simulink model "Excavator_Complete"  (R2026a)
settings: Solver=ode23t  StopTime=stopTime  MaxStep=Ts  AbsTol=1e-3
PostLoadFcn:
  | set_param(bdroot,'IgnoredZcDiagnostic','none');
  | Excavator_Test_Scenario_Select('loadedBucketDigCycle');
model workspace: external: MAT-File ExcavatorAssemblyDataStruct.mat (data not in the file)
undefined symbols (not defined in the file or in its folder): AToBRegOrificeVector, AToTOrificeVector, BiPOrificeVector, BoomC, boomHEArea, boomREArea, boomUpMaxQ, boomValve, BToTOrificeVector, BucketC, bucketCloseMaxQ, bucketOpenMaxQ, BucketR, bucketValve, fluids, gravity, LeftBoomR, materialWeight, maxPumpDisp, minPumpDisp, nominalEngineSpeed, P28Assembly, PToAOrificeVector, PToBOrificeVector, pumpCmdNegRateLimit, pumpCmdPosRateLimit, RightBoomR, startDiggingZPos, StickC, stickInMaxQ, stickOutMaxQ, StickR, stickValve, SwingC, swingDisplacement, swingHighSpeedThreshold, swingMaxQ, SwingR, swingSpeedQGain, swingValve, valveCmdNegRateLimit, valveCmdPosRateLimit, velocityToYForceGain, X, Y, yForceMax, yForceToZForceGain, Z, zForceMax
libraries: fl_lib x89, sm_lib x80, SimscapeFluids_lib x78, nesl_utility x50, simulink_extras x11, Excavator_Parts_Lib x6, simulink x2, SignalEditorBlockLib x1
(part 7 of 7)

== system Excavator_Complete/Excavator/Hydraulics/ValveBlocks/RightValveBlock/Bucket Valve ==
  AtoT : SimscapeFluids_lib/Isothermal Liquid/Valves & Orifices/Orifices/Orifice (IL)  orifice_type=foundation.enum.constant_variable.variable  constant_orifice_spec=fluids.isothermal_liquid.valves_orifices.orifices.enum.constant_orifice_spec.area  variable_orifice_spec=fluids.isothermal_liquid.valves_orifices.orifices.enum.orifice_spec.table1D_area_opening  orifice_area_constant=1e-3 m^2  p_diff_TLU_constant=[-4, -3, -2, -1, -.5, 0, .5, 1, 2, 3, 4] MPa  vol_flow_TLU_constant=[-2.44, -2.12, -1.68, -1.22, -.84, 0, .85, 1.21, 1.7, 2.09, 2.41] .* 1e-3 m^3/s  S_min=1e-10 m  del_S=0.005 m  open_orientation=fluids.isothermal_liquid.valves_orifices.orifices.enum.orifice_orientation.positive  area_max=0.5e-4 m^2  area_leak=1e-12 m^2  S_TLU=valveData.spoolPosVector mm  orifice_area_TLU=valveData.AtoTOrificeAreaVector mm^2  area=inf m^2  Cd=0.7  Re_c=150  smoothing_factor=0  pressure_recovery=simscape.enum.onoff.off  S_vol_flow_TLU=AToTOrificeVector - 1000*(0) mm  p_diff_TLU=[-10000000, -5000000, -2000000, 2000000, 5000000, 10000000] Pa  vol_flow_TLU=[-1e-07, -7.0711e-08, -4.4721e-08, 4.4721e-08, 7.0711e-08, 1e-07; -2.0352e-05, -1.4391e-05, -9.1017e-06, 9.1017e-06, 1.4391e-05, 2.0352e-05; -.0040736, -.0028805, -.0018218, .0018218, .0028805, .0040736; -.011438, -.0080879, -.0051152, .0051152, .0080879, .011438; -.034356, -.024293, -.015364, .015364, .024293, .034356] m^3/s
  BiPOrifice : SimscapeFluids_lib/Isothermal Liquid/Valves & Orifices/Orifices/Orifice (IL)  orifice_type=foundation.enum.constant_variable.variable  constant_orifice_spec=fluids.isothermal_liquid.valves_orifices.orifices.enum.constant_orifice_spec.area  variable_orifice_spec=fluids.isothermal_liquid.valves_orifices.orifices.enum.orifice_spec.table1D_area_opening  orifice_area_constant=1e-3 m^2  p_diff_TLU_constant=[-4, -3, -2, -1, -.5, 0, .5, 1, 2, 3, 4] MPa  vol_flow_TLU_constant=[-2.44, -2.12, -1.68, -1.22, -.84, 0, .85, 1.21, 1.7, 2.09, 2.41] .* 1e-3 m^3/s  S_min=1e-10 m  del_S=0.005 m  open_orientation=fluids.isothermal_liquid.valves_orifices.orifices.enum.orifice_orientation.positive  area_max=0.5e-4 m^2  area_leak=1e-12 m^2  S_TLU=valveData.spoolPosVector mm  orifice_area_TLU=valveData.BiPOrificeAreaVector mm^2  area=inf m^2  Cd=0.7  Re_c=150  smoothing_factor=0  pressure_recovery=simscape.enum.onoff.off  S_vol_flow_TLU=BiPOrificeVector - 1000*(0) mm  p_diff_TLU=[-10000000, -5000000, -2000000, 2000000, 5000000, 10000000] Pa  vol_flow_TLU=[-1e-07, -7.0711e-08, -4.4721e-08, 4.4721e-08, 7.0711e-08, 1e-07; -2.0352e-05, -1.4391e-05, -9.1017e-06, 9.1017e-06, 1.4391e-05, 2.0352e-05; -.0040736, -.0028805, -.0018218, .0018218, .0028805, .0040736; -.011438, -.0080879, -.0051152, .0051152, .0080879, .011438; -.034356, -.024293, -.015364, .015364, .024293, .034356] m^3/s
  BtoT : SimscapeFluids_lib/Isothermal Liquid/Valves & Orifices/Orifices/Orifice (IL)  orifice_type=foundation.enum.constant_variable.variable  constant_orifice_spec=fluids.isothermal_liquid.valves_orifices.orifices.enum.constant_orifice_spec.area  variable_orifice_spec=fluids.isothermal_liquid.valves_orifices.orifices.enum.orifice_spec.table1D_area_opening  orifice_area_constant=1e-3 m^2  p_diff_TLU_constant=[-4, -3, -2, -1, -.5, 0, .5, 1, 2, 3, 4] MPa  vol_flow_TLU_constant=[-2.44, -2.12, -1.68, -1.22, -.84, 0, .85, 1.21, 1.7, 2.09, 2.41] .* 1e-3 m^3/s  S_min=1e-10 m  del_S=0.005 m  open_orientation=fluids.isothermal_liquid.valves_orifices.orifices.enum.orifice_orientation.positive  area_max=0.5e-4 m^2  area_leak=1e-12 m^2  S_TLU=valveData.spoolPosVector mm  orifice_area_TLU=valveData.BtoTOrificeAreaVector mm^2  area=inf m^2  Cd=0.7  Re_c=150  smoothing_factor=0  pressure_recovery=simscape.enum.onoff.off  S_vol_flow_TLU=BToTOrificeVector - 1000*(0) mm  p_diff_TLU=[-10000000, -5000000, -2000000, 2000000, 5000000, 10000000] Pa  vol_flow_TLU=[-1e-07, -7.0711e-08, -4.4721e-08, 4.4721e-08, 7.0711e-08, 1e-07; -2.0352e-05, -1.4391e-05, -9.1017e-06, 9.1017e-06, 1.4391e-05, 2.0352e-05; -.0040736, -.0028805, -.0018218, .0018218, .0028805, .0040736; -.011438, -.0080879, -.0051152, .0051152, .0080879, .011438; -.034356, -.024293, -.015364, .015364, .024293, .034356] m^3/s
  PS Abs : fl_lib/Physical Signals/Nonlinear Operators/PS Abs  ZeroCross=true
  PS Gain1 : fl_lib/Physical Signals/Functions/PS Gain  gain=-1
  PtoA : SimscapeFluids_lib/Isothermal Liquid/Valves & Orifices/Orifices/Orifice (IL)  orifice_type=foundation.enum.constant_variable.variable  constant_orifice_spec=fluids.isothermal_liquid.valves_orifices.orifices.enum.constant_orifice_spec.area  variable_orifice_spec=fluids.isothermal_liquid.valves_orifices.orifices.enum.orifice_spec.table1D_area_opening  orifice_area_constant=1e-3 m^2  p_diff_TLU_constant=[-4, -3, -2, -1, -.5, 0, .5, 1, 2, 3, 4] MPa  vol_flow_TLU_constant=[-2.44, -2.12, -1.68, -1.22, -.84, 0, .85, 1.21, 1.7, 2.09, 2.41] .* 1e-3 m^3/s  S_min=1e-10 m  del_S=0.005 m  open_orientation=fluids.isothermal_liquid.valves_orifices.orifices.enum.orifice_orientation.positive  area_max=0.5e-4 m^2  area_leak=1e-12 m^2  S_TLU=valveData.spoolPosVector mm  orifice_area_TLU=valveData.PtoAOrificeAreaVector mm^2  area=inf m^2  Cd=0.7  Re_c=150  smoothing_factor=0  pressure_recovery=simscape.enum.onoff.off  S_vol_flow_TLU=PToAOrificeVector - 1000*(0) mm  p_diff_TLU=[-10000000, -5000000, -2000000, 2000000, 5000000, 10000000] Pa  vol_flow_TLU=[-1e-07, -7.0711e-08, -4.4721e-08, 4.4721e-08, 7.0711e-08, 1e-07; -2.0352e-05, -1.4391e-05, -9.1017e-06, 9.1017e-06, 1.4391e-05, 2.0352e-05; -.0040736, -.0028805, -.0018218, .0018218, .0028805, .0040736; -.011438, -.0080879, -.0051152, .0051152, .0080879, .011438; -.034356, -.024293, -.015364, .015364, .024293, .034356] m^3/s
  PtoB : SimscapeFluids_lib/Isothermal Liquid/Valves & Orifices/Orifices/Orifice (IL)  orifice_type=foundation.enum.constant_variable.variable  constant_orifice_spec=fluids.isothermal_liquid.valves_orifices.orifices.enum.constant_orifice_spec.area  variable_orifice_spec=fluids.isothermal_liquid.valves_orifices.orifices.enum.orifice_spec.table1D_area_opening  orifice_area_constant=1e-3 m^2  p_diff_TLU_constant=[-4, -3, -2, -1, -.5, 0, .5, 1, 2, 3, 4] MPa  vol_flow_TLU_constant=[-2.44, -2.12, -1.68, -1.22, -.84, 0, .85, 1.21, 1.7, 2.09, 2.41] .* 1e-3 m^3/s  S_min=1e-10 m  del_S=0.005 m  open_orientation=fluids.isothermal_liquid.valves_orifices.orifices.enum.orifice_orientation.positive  area_max=0.5e-4 m^2  area_leak=1e-12 m^2  S_TLU=valveData.spoolPosVector mm  orifice_area_TLU=valveData.PtoBOrificeAreaVector mm^2  area=inf m^2  Cd=0.7  Re_c=150  smoothing_factor=0  pressure_recovery=simscape.enum.onoff.off  S_vol_flow_TLU=PToBOrificeVector - 1000*(0) mm  p_diff_TLU=[-10000000, -5000000, -2000000, 2000000, 5000000, 10000000] Pa  vol_flow_TLU=[-1e-07, -7.0711e-08, -4.4721e-08, 4.4721e-08, 7.0711e-08, 1e-07; -2.0352e-05, -1.4391e-05, -9.1017e-06, 9.1017e-06, 1.4391e-05, 2.0352e-05; -.0040736, -.0028805, -.0018218, .0018218, .0028805, .0040736; -.011438, -.0080879, -.0051152, .0051152, .0080879, .011438; -.034356, -.024293, -.015364, .015364, .024293, .034356] m^3/s
  S : PMIOPort  Side=Left
  P : PMIOPort  Port=2  Side=Left
  T : PMIOPort  Port=3  Side=Left
  BiPIn : PMIOPort  Port=4  Side=Left
  A : PMIOPort  Port=5  Side=Right
  B : PMIOPort  Port=6  Side=Right
  BiPOut : PMIOPort  Port=7  Side=Right
  connections:
  BtoT/LConn2 -- PtoA/LConn2 -- PS Gain1/RConn1
  BiPOrifice/LConn2 -- PS Abs/RConn1
  S/RConn1 -- PtoB/LConn2 -- AtoT/LConn2 -- PS Gain1/LConn1 -- PS Abs/LConn1
  T/RConn1 -- BtoT/RConn1 -- AtoT/RConn1
  BiPOrifice/RConn1 -- BiPOut/RConn1
  BiPOrifice/LConn1 -- BiPIn/RConn1
  PtoA/RConn1 -- A/RConn1 -- AtoT/LConn1
  PtoB/LConn1 -- P/RConn1 -- PtoA/LConn1
  PtoB/RConn1 -- BtoT/LConn1 -- B/RConn1

== system Excavator_Complete/Excavator/Hydraulics/ValveBlocks/RightValveBlock/Cmd to Spool Pos ==
  Cmds : Inport
  Bus Selector : BusSelector  OutputSignals=BMSpoolPos,SKSpoolPos,BTSpoolPos
  Simulink-PS Converter : nesl_utility/Simulink-PS Converter  PhysicalDomain=network_engine_domain  SubClassName=ps_input  LeftPortType=input  RightPortType=output  PseudoPeriodic=off  Frequencies=[]  NoiseDistribution=none  NoiseParameters=[]  Unit=mm  AffineConversion=off  FilteringAndDerivatives=provide  SimscapeFilterOrder=1  InputFilterTimeConstant=0.001  UdotUserProvided=0
  Simulink-PS Converter1 : nesl_utility/Simulink-PS Converter  PhysicalDomain=network_engine_domain  SubClassName=ps_input  LeftPortType=input  RightPortType=output  PseudoPeriodic=off  Frequencies=[]  NoiseDistribution=none  NoiseParameters=[]  Unit=mm  AffineConversion=off  FilteringAndDerivatives=provide  SimscapeFilterOrder=1  InputFilterTimeConstant=0.001  UdotUserProvided=0
  Simulink-PS Converter2 : nesl_utility/Simulink-PS Converter  PhysicalDomain=network_engine_domain  SubClassName=ps_input  LeftPortType=input  RightPortType=output  PseudoPeriodic=off  Frequencies=[]  NoiseDistribution=none  NoiseParameters=[]  Unit=mm  AffineConversion=off  FilteringAndDerivatives=provide  SimscapeFilterOrder=1  InputFilterTimeConstant=0.001  UdotUserProvided=0
  BMPos : PMIOPort  Side=Right
  SKPos : PMIOPort  Port=2  Side=Right
  BTPos : PMIOPort  Port=3  Side=Right
  wires:
  Bus Selector/1 -> Simulink-PS Converter/1  "<BMSpoolPos>"
  Bus Selector/3 -> Simulink-PS Converter2/1  "<BTSpoolPos>"
  Bus Selector/2 -> Simulink-PS Converter1/1  "<SKSpoolPos>"
  Cmds/1 -> Bus Selector/1
  connections:
  Simulink-PS Converter/RConn1 -- BMPos/RConn1
  Simulink-PS Converter1/RConn1 -- SKPos/RConn1
  Simulink-PS Converter2/RConn1 -- BTPos/RConn1

== system Excavator_Complete/Excavator/Hydraulics/ValveBlocks/RightValveBlock/Stick Valve ==
  AtoT : SimscapeFluids_lib/Isothermal Liquid/Valves & Orifices/Orifices/Orifice (IL)  orifice_type=foundation.enum.constant_variable.variable  constant_orifice_spec=fluids.isothermal_liquid.valves_orifices.orifices.enum.constant_orifice_spec.area  variable_orifice_spec=fluids.isothermal_liquid.valves_orifices.orifices.enum.orifice_spec.table1D_area_opening  orifice_area_constant=1e-3 m^2  p_diff_TLU_constant=[-4, -3, -2, -1, -.5, 0, .5, 1, 2, 3, 4] MPa  vol_flow_TLU_constant=[-2.44, -2.12, -1.68, -1.22, -.84, 0, .85, 1.21, 1.7, 2.09, 2.41] .* 1e-3 m^3/s  S_min=1e-10 m  del_S=0.005 m  open_orientation=fluids.isothermal_liquid.valves_orifices.orifices.enum.orifice_orientation.positive  area_max=0.5e-4 m^2  area_leak=1e-12 m^2  S_TLU=valveData.spoolPosVector mm  orifice_area_TLU=valveData.AtoTOrificeAreaVector mm^2  area=inf m^2  Cd=0.7  Re_c=150  smoothing_factor=0  pressure_recovery=simscape.enum.onoff.off  S_vol_flow_TLU=AToTOrificeVector - 1000*(0) mm  p_diff_TLU=[-10000000, -5000000, -2000000, 2000000, 5000000, 10000000] Pa  vol_flow_TLU=[-1e-07, -7.0711e-08, -4.4721e-08, 4.4721e-08, 7.0711e-08, 1e-07; -2.0352e-05, -1.4391e-05, -9.1017e-06, 9.1017e-06, 1.4391e-05, 2.0352e-05; -.0040736, -.0028805, -.0018218, .0018218, .0028805, .0040736; -.011438, -.0080879, -.0051152, .0051152, .0080879, .011438; -.034356, -.024293, -.015364, .015364, .024293, .034356] m^3/s
  BiPOrifice : SimscapeFluids_lib/Isothermal Liquid/Valves & Orifices/Orifices/Orifice (IL)  orifice_type=foundation.enum.constant_variable.variable  constant_orifice_spec=fluids.isothermal_liquid.valves_orifices.orifices.enum.constant_orifice_spec.area  variable_orifice_spec=fluids.isothermal_liquid.valves_orifices.orifices.enum.orifice_spec.table1D_area_opening  orifice_area_constant=1e-3 m^2  p_diff_TLU_constant=[-4, -3, -2, -1, -.5, 0, .5, 1, 2, 3, 4] MPa  vol_flow_TLU_constant=[-2.44, -2.12, -1.68, -1.22, -.84, 0, .85, 1.21, 1.7, 2.09, 2.41] .* 1e-3 m^3/s  S_min=1e-10 m  del_S=0.005 m  open_orientation=fluids.isothermal_liquid.valves_orifices.orifices.enum.orifice_orientation.positive  area_max=0.5e-4 m^2  area_leak=1e-12 m^2  S_TLU=valveData.spoolPosVector mm  orifice_area_TLU=valveData.BiPOrificeAreaVector mm^2  area=inf m^2  Cd=0.7  Re_c=150  smoothing_factor=0  pressure_recovery=simscape.enum.onoff.off  S_vol_flow_TLU=BiPOrificeVector - 1000*(0) mm  p_diff_TLU=[-10000000, -5000000, -2000000, 2000000, 5000000, 10000000] Pa  vol_flow_TLU=[-1e-07, -7.0711e-08, -4.4721e-08, 4.4721e-08, 7.0711e-08, 1e-07; -2.0352e-05, -1.4391e-05, -9.1017e-06, 9.1017e-06, 1.4391e-05, 2.0352e-05; -.0040736, -.0028805, -.0018218, .0018218, .0028805, .0040736; -.011438, -.0080879, -.0051152, .0051152, .0080879, .011438; -.034356, -.024293, -.015364, .015364, .024293, .034356] m^3/s
  BtoARegen : SimscapeFluids_lib/Isothermal Liquid/Valves & Orifices/Orifices/Orifice (IL)  orifice_type=foundation.enum.constant_variable.variable  constant_orifice_spec=fluids.isothermal_liquid.valves_orifices.orifices.enum.constant_orifice_spec.area  variable_orifice_spec=fluids.isothermal_liquid.valves_orifices.orifices.enum.orifice_spec.table1D_area_opening  orifice_area_constant=1e-3 m^2  p_diff_TLU_constant=[-4, -3, -2, -1, -.5, 0, .5, 1, 2, 3, 4] MPa  vol_flow_TLU_constant=[-2.44, -2.12, -1.68, -1.22, -.84, 0, .85, 1.21, 1.7, 2.09, 2.41] .* 1e-3 m^3/s  S_min=1e-10 m  del_S=0.005 m  open_orientation=fluids.isothermal_liquid.valves_orifices.orifices.enum.orifice_orientation.positive  area_max=0.5e-4 m^2  area_leak=1e-12 m^2  S_TLU=valveData.spoolPosVector mm  orifice_area_TLU=valveData.BtoARegOrificeAreaVector mm^2  area=inf m^2  Cd=0.7  Re_c=150  smoothing_factor=0  pressure_recovery=simscape.enum.onoff.off  S_vol_flow_TLU=AToBRegOrificeVector - 1000*(0) mm  p_diff_TLU=[-10000000, -5000000, -2000000, 2000000, 5000000, 10000000] Pa  vol_flow_TLU=[-1e-07, -7.0711e-08, -4.4721e-08, 4.4721e-08, 7.0711e-08, 1e-07; -2.0352e-05, -1.4391e-05, -9.1017e-06, 9.1017e-06, 1.4391e-05, 2.0352e-05; -.0040736, -.0028805, -.0018218, .0018218, .0028805, .0040736; -.011438, -.0080879, -.0051152, .0051152, .0080879, .011438; -.034356, -.024293, -.015364, .015364, .024293, .034356] m^3/s
  BtoT : SimscapeFluids_lib/Isothermal Liquid/Valves & Orifices/Orifices/Orifice (IL)  orifice_type=foundation.enum.constant_variable.variable  constant_orifice_spec=fluids.isothermal_liquid.valves_orifices.orifices.enum.constant_orifice_spec.area  variable_orifice_spec=fluids.isothermal_liquid.valves_orifices.orifices.enum.orifice_spec.table1D_area_opening  orifice_area_constant=1e-3 m^2  p_diff_TLU_constant=[-4, -3, -2, -1, -.5, 0, .5, 1, 2, 3, 4] MPa  vol_flow_TLU_constant=[-2.44, -2.12, -1.68, -1.22, -.84, 0, .85, 1.21, 1.7, 2.09, 2.41] .* 1e-3 m^3/s  S_min=1e-10 m  del_S=0.005 m  open_orientation=fluids.isothermal_liquid.valves_orifices.orifices.enum.orifice_orientation.positive  area_max=0.5e-4 m^2  area_leak=1e-12 m^2  S_TLU=valveData.spoolPosVector mm  orifice_area_TLU=valveData.BtoTOrificeAreaVector mm^2  area=inf m^2  Cd=0.7  Re_c=150  smoothing_factor=0  pressure_recovery=simscape.enum.onoff.off  S_vol_flow_TLU=BToTOrificeVector - 1000*(0) mm  p_diff_TLU=[-10000000, -5000000, -2000000, 2000000, 5000000, 10000000] Pa  vol_flow_TLU=[-1e-07, -7.0711e-08, -4.4721e-08, 4.4721e-08, 7.0711e-08, 1e-07; -2.0352e-05, -1.4391e-05, -9.1017e-06, 9.1017e-06, 1.4391e-05, 2.0352e-05; -.0040736, -.0028805, -.0018218, .0018218, .0028805, .0040736; -.011438, -.0080879, -.0051152, .0051152, .0080879, .011438; -.034356, -.024293, -.015364, .015364, .024293, .034356] m^3/s
  PS Abs : fl_lib/Physical Signals/Nonlinear Operators/PS Abs  ZeroCross=true
  PS Gain1 : fl_lib/Physical Signals/Functions/PS Gain  gain=-1
  PtoA : SimscapeFluids_lib/Isothermal Liquid/Valves & Orifices/Orifices/Orifice (IL)  orifice_type=foundation.enum.constant_variable.variable  constant_orifice_spec=fluids.isothermal_liquid.valves_orifices.orifices.enum.constant_orifice_spec.area  variable_orifice_spec=fluids.isothermal_liquid.valves_orifices.orifices.enum.orifice_spec.table1D_area_opening  orifice_area_constant=1e-3 m^2  p_diff_TLU_constant=[-4, -3, -2, -1, -.5, 0, .5, 1, 2, 3, 4] MPa  vol_flow_TLU_constant=[-2.44, -2.12, -1.68, -1.22, -.84, 0, .85, 1.21, 1.7, 2.09, 2.41] .* 1e-3 m^3/s  S_min=1e-10 m  del_S=0.005 m  open_orientation=fluids.isothermal_liquid.valves_orifices.orifices.enum.orifice_orientation.positive  area_max=0.5e-4 m^2  area_leak=1e-12 m^2  S_TLU=valveData.spoolPosVector mm  orifice_area_TLU=valveData.PtoAOrificeAreaVector mm^2  area=inf m^2  Cd=0.7  Re_c=150  smoothing_factor=0  pressure_recovery=simscape.enum.onoff.off  S_vol_flow_TLU=PToAOrificeVector - 1000*(0) mm  p_diff_TLU=[-10000000, -5000000, -2000000, 2000000, 5000000, 10000000] Pa  vol_flow_TLU=[-1e-07, -7.0711e-08, -4.4721e-08, 4.4721e-08, 7.0711e-08, 1e-07; -2.0352e-05, -1.4391e-05, -9.1017e-06, 9.1017e-06, 1.4391e-05, 2.0352e-05; -.0040736, -.0028805, -.0018218, .0018218, .0028805, .0040736; -.011438, -.0080879, -.0051152, .0051152, .0080879, .011438; -.034356, -.024293, -.015364, .015364, .024293, .034356] m^3/s
  PtoB : SimscapeFluids_lib/Isothermal Liquid/Valves & Orifices/Orifices/Orifice (IL)  orifice_type=foundation.enum.constant_variable.variable  constant_orifice_spec=fluids.isothermal_liquid.valves_orifices.orifices.enum.constant_orifice_spec.area  variable_orifice_spec=fluids.isothermal_liquid.valves_orifices.orifices.enum.orifice_spec.table1D_area_opening  orifice_area_constant=1e-3 m^2  p_diff_TLU_constant=[-4, -3, -2, -1, -.5, 0, .5, 1, 2, 3, 4] MPa  vol_flow_TLU_constant=[-2.44, -2.12, -1.68, -1.22, -.84, 0, .85, 1.21, 1.7, 2.09, 2.41] .* 1e-3 m^3/s  S_min=1e-10 m  del_S=0.005 m  open_orientation=fluids.isothermal_liquid.valves_orifices.orifices.enum.orifice_orientation.positive  area_max=0.5e-4 m^2  area_leak=1e-12 m^2  S_TLU=valveData.spoolPosVector mm  orifice_area_TLU=valveData.PtoBOrificeAreaVector mm^2  area=inf m^2  Cd=0.7  Re_c=150  smoothing_factor=0  pressure_recovery=simscape.enum.onoff.off  S_vol_flow_TLU=PToBOrificeVector - 1000*(0) mm  p_diff_TLU=[-10000000, -5000000, -2000000, 2000000, 5000000, 10000000] Pa  vol_flow_TLU=[-1e-07, -7.0711e-08, -4.4721e-08, 4.4721e-08, 7.0711e-08, 1e-07; -2.0352e-05, -1.4391e-05, -9.1017e-06, 9.1017e-06, 1.4391e-05, 2.0352e-05; -.0040736, -.0028805, -.0018218, .0018218, .0028805, .0040736; -.011438, -.0080879, -.0051152, .0051152, .0080879, .011438; -.034356, -.024293, -.015364, .015364, .024293, .034356] m^3/s
  StickRegenCV : SimscapeFluids_lib/Isothermal Liquid/Valves & Orifices/Directional Control Valves/Check Valve (IL)  opening_spec=2*(fluids.isothermal_liquid.valves_orifices.enum.opening_spec.linear)-1  pressure_control_spec=fluids.isothermal_liquid.valves_orifices.enum.pressure_control_spec.dp  p_crack_differential=valveData.checkValveCrackingPrDiff bar  p_crack_gauge=0.1 MPa  press_max_differential=valveData.checkValveMaxOpeningPrDiff bar  press_max_gauge=0.2 MPa  area_max=valveData.checkValveMaxOpeningArea mm^2  area_leak=valveData.checkValveLeakageArea mm^2  p_diff_TLU=[0.01 : 0.01 : 0.1] MPa  valve_area_TLU=[1e-10, 1e-05, 2e-05, 3e-05, 4e-05, 5e-05, 6e-05, 7.5e-05, 8.5e-05, .0001] m^2  vol_flow_TLU=[.000358, .045, .11, .191, .284, .39, .505, .63, .764, .905] .* 1e-3 m^3/s  area=inf m^2  Cd=0.7  Re_c=150  smoothing_factor=0.1  pressure_recovery=simscape.enum.onoff.off  opening_dynamics=simscape.enum.onoff.off  tau=0.1 s
  Volume Regen Valve : fl_lib/Isothermal Liquid/Elements/Constant Volume Chamber (IL)  volume=vcVol m^3  p_I_specify=on  p_I_priority=High  p_I=initStickHEPr bar  p_I_nominal_specify=off  p_I_nominal_value=1  p_I_nominal_unit=MPa
  S : PMIOPort  Side=Left
  P : PMIOPort  Port=2  Side=Left
  T : PMIOPort  Port=3  Side=Left
  BiPIn : PMIOPort  Port=4  Side=Left
  A : PMIOPort  Port=5  Side=Right
  B : PMIOPort  Port=6  Side=Right
  BiPOut : PMIOPort  Port=7  Side=Right
  connections:
  BtoT/LConn2 -- PS Gain1/RConn1 -- BtoARegen/LConn2 -- PtoA/LConn2
  BiPOrifice/LConn2 -- PS Abs/RConn1
  AtoT/LConn2 -- PS Gain1/LConn1 -- PS Abs/LConn1 -- S/RConn1 -- PtoB/LConn2
  BtoARegen/RConn1 -- StickRegenCV/LConn1 -- Volume Regen Valve/LConn1
  T/RConn1 -- BtoT/RConn1 -- AtoT/RConn1
  BiPOrifice/RConn1 -- BiPOut/RConn1
  BiPOrifice/LConn1 -- BiPIn/RConn1
  PtoA/RConn1 -- A/RConn1 -- StickRegenCV/RConn1 -- AtoT/LConn1
  P/RConn1 -- PtoB/LConn1 -- PtoA/LConn1
  BtoARegen/LConn1 -- PtoB/RConn1 -- BtoT/LConn1 -- B/RConn1

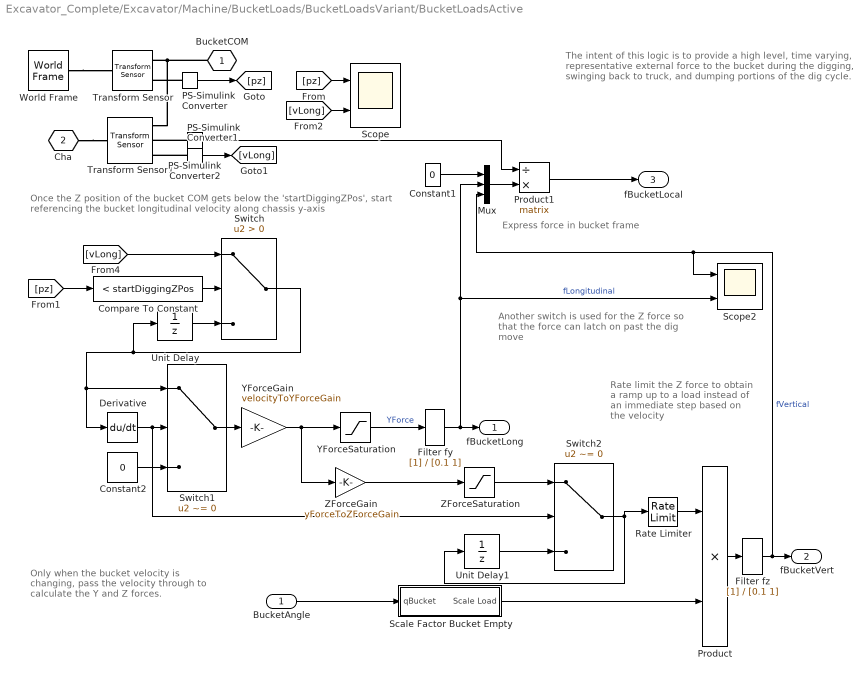
== system Excavator_Complete/Excavator/Machine/BucketLoads/BucketLoadsVariant/BucketLoadsActive ==
  note: Express force in bucket frame
  note: Once the Z position of the bucket COM gets below the 'startDiggingZPos', start referencing the bucket longitudinal velocity along chassis y-axis
  note: Only when the bucket velocity is changing, pass the velocity through to calculate the Y and Z forces.
  note: Another switch is used for the Z force so that the force can latch on past the dig move
  note: Rate limit the Z force to obtain a ramp up to a load instead of an immediate step based on the velocity
  note: The intent of this logic is to provide a high level, time varying, representative external force to the bucket during the digging, swinging back to truck, and dumping portions of the dig cycle.
  BucketAngle : Inport
  Compare To Constant : simulink/Logic and Bit Operations/Compare To Constant  relop=<  const=startDiggingZPos  OutDataTypeStr=boolean
  Constant1 : Constant  Value=0
  Constant2 : Constant  Value=0
  Derivative : Derivative
  Filter fy : TransferFcn  Denominator=[0.1 1]
  Filter fz : TransferFcn  Denominator=[0.1 1]
  Mux : Mux  Inputs=3
  PS-Simulink Converter : nesl_utility/PS-Simulink Converter  PhysicalDomain=network_engine_domain  SubClassName=ps_output  LeftPortType=input  RightPortType=output  PseudoPeriodic=off  Frequencies=[]  VectorFormat=inherit  Unit=mm  AffineConversion=off
  PS-Simulink Converter1 : nesl_utility/PS-Simulink Converter  PhysicalDomain=network_engine_domain  SubClassName=ps_output  LeftPortType=input  RightPortType=output  PseudoPeriodic=off  Frequencies=[]  VectorFormat=inherit  Unit=mm/s  AffineConversion=off
  PS-Simulink Converter2 : nesl_utility/PS-Simulink Converter  PhysicalDomain=network_engine_domain  SubClassName=ps_output  LeftPortType=input  RightPortType=output  PseudoPeriodic=off  Frequencies=[]  VectorFormat=inherit  Unit=inherit  AffineConversion=off
  Product : Product
  Product1 : Product  Inputs=/*  Multiplication=Matrix(*)
  Rate Limiter : RateLimiter  RisingSlewLimit=750  FallingSlewLimit=-80  SampleTimeMode=inherited
  Scale Factor Bucket Empty : Subsystem
  Scope : Scope  NumInputPorts=2
      settings: ActiveDisplayYMinimum=-4867.9057  ActiveDisplayYMaximum=4889.74505
  Scope2 : Scope  NumInputPorts=2
      settings: ActiveDisplayYMinimum=-174.28167  ActiveDisplayYMaximum=248.19229  DataLoggingVariableName=ScopeData3
  Switch : Switch  Criteria=u2 > Threshold  SaturateOnIntegerOverflow=off  InputSameDT=off
  Switch1 : Switch  Criteria=u2 ~= 0  ZeroCross=off  SaturateOnIntegerOverflow=off  InputSameDT=off
  Switch2 : Switch  Criteria=u2 ~= 0  ZeroCross=off  SaturateOnIntegerOverflow=off  InputSameDT=off
  Transform Sensor : sm_lib/Frames and Transforms/Transform Sensor  MeasurementFrame=World  RotationSequence=XYX  SenseAngle=off  SenseAxis=off  SenseQ=off  SenseR=off  SenseRotationSequence=off  SenseOmegaX=off  SenseOmegaY=off  SenseOmegaZ=off  SenseOmega=off  SenseQDot=off  SenseRDot=off  SenseRotationSequenceDot=off  SenseAlphaX=off  SenseAlphaY=off  SenseAlphaZ=off  SenseAlpha=off  SenseQDDot=off  SenseRDDot=off  SenseX=off  SenseY=off  SenseZ=on  SenseXYZ=off  SenseRad=off  SenseAzim=off  SenseDist=off  SenseInc=off  SenseXDot=off  SenseYDot=off  SenseZDot=off  SenseXYZDot=off  SenseRadDot=off  SenseAzimDot=off  SenseDistDot=off  SenseIncDot=off  SenseXDDot=off  SenseYDDot=off  SenseZDDot=off  SenseXYZDDot=off  SenseRadDDot=off  SenseAzimDDot=off  SenseDistDDot=off  SenseIncDDot=off
  Transform Sensor1 : sm_lib/Frames and Transforms/Transform Sensor  MeasurementFrame=Base  RotationSequence=ZYX  SenseAngle=off  SenseAxis=off  SenseQ=off  SenseR=on  SenseRotationSequence=off  SenseOmegaX=off  SenseOmegaY=off  SenseOmegaZ=off  SenseOmega=off  SenseQDot=off  SenseRDot=off  SenseRotationSequenceDot=off  SenseAlphaX=off  SenseAlphaY=off  SenseAlphaZ=off  SenseAlpha=off  SenseQDDot=off  SenseRDDot=off  SenseX=off  SenseY=off  SenseZ=off  SenseXYZ=off  SenseRad=off  SenseAzim=off  SenseDist=off  SenseInc=off  SenseXDot=off  SenseYDot=on  SenseZDot=off  SenseXYZDot=off  SenseRadDot=off  SenseAzimDot=off  SenseDistDot=off  SenseIncDot=off  SenseXDDot=off  SenseYDDot=off  SenseZDDot=off  SenseXYZDDot=off  SenseRadDDot=off  SenseAzimDDot=off  SenseDistDDot=off  SenseIncDDot=off
  Unit Delay : UnitDelay  SampleTime=-1
  Unit Delay1 : UnitDelay  SampleTime=-1
  World Frame : sm_lib/Frames and Transforms/World Frame
  YForceGain : Gain  Gain=velocityToYForceGain
  YForceSaturation : Saturate  UpperLimit=yForceMax  LowerLimit=0
  ZForceGain : Gain  Gain=yForceToZForceGain
  ZForceSaturation : Saturate  UpperLimit=-materialWeight  LowerLimit=-zForceMax  ZeroCross=off
  BucketCOM : PMIOPort  Side=Left
  Cha : PMIOPort  Port=2  Side=Left
  fBucketLong : Outport
  fBucketVert : Outport  Port=2
  fBucketLocal : Outport  Port=3
  wires:
  ZForceSaturation/1 -> Switch2/1
  Unit Delay1/1 -> Switch2/3
  Filter fy/1 -> Mux/2, Scope2/2, fBucketLong/1  "fLongitudinal"
  Compare To Constant/1 -> Switch/2
  Unit Delay/1 -> Switch/3
  Switch1/1 -> YForceGain/1
  Switch/1 -> Switch1/1, Derivative/1, Unit Delay/1
  PS-Simulink Converter/1 -> [pz]
  PS-Simulink Converter1/1 -> [vLong]
  Constant2/1 -> Switch1/3
  Switch2/1 -> Rate Limiter/1, Unit Delay1/1
  Rate Limiter/1 -> Product/1
  Filter fz/1 -> fBucketVert/1, Mux/3, Scope2/1  "fVertical"
  ZForceGain/1 -> ZForceSaturation/1
  Derivative/1 -> Switch2/2, Switch1/2
  YForceGain/1 -> YForceSaturation/1, ZForceGain/1
  YForceSaturation/1 -> Filter fy/1  "YForce"
  Product/1 -> Filter fz/1
  Constant1/1 -> Mux/1
  PS-Simulink Converter2/1 -> Product1/1
  Product1/1 -> fBucketLocal/1
  Mux/1 -> Product1/2
  [pz] -> Scope/1
  [pz] -> Compare To Constant/1
  [vLong] -> Scope/2
  [vLong] -> Switch/1
  BucketAngle/1 -> Scale Factor Bucket Empty/1(qBucket)
  Scale Factor Bucket Empty/1(Scale Load) -> Product/2
  connections:
  PS-Simulink Converter1/LConn1 -- Transform Sensor1/RConn3
  PS-Simulink Converter/LConn1 -- Transform Sensor/RConn2
  World Frame/RConn1 -- Transform Sensor/LConn1
  BucketCOM/RConn1 -- Transform Sensor1/RConn1 -- Transform Sensor/RConn1
  Cha/RConn1 -- Transform Sensor1/LConn1
  PS-Simulink Converter2/LConn1 -- Transform Sensor1/RConn2

== system Excavator_Complete/Excavator/Machine/BucketLoads/BucketLoadsVariant/BucketLoadsInactive ==
  BucketAngle : Inport
  Constant : Constant  Value=[0 0 0]
  Constant1 : Constant  Value=0
  Constant2 : Constant  Value=0
  Terminator : Terminator
  BucketCOM : PMIOPort  Side=Left
  Cha : PMIOPort  Port=2  Side=Left
  fBucketLong : Outport
  fBucketVert : Outport  Port=2
  fBucketLocal : Outport  Port=3
  wires:
  Constant/1 -> fBucketLocal/1
  BucketAngle/1 -> Terminator/1
  Constant1/1 -> fBucketLong/1
  Constant2/1 -> fBucketVert/1

== system Excavator_Complete/Excavator/Machine/BucketLoads/BucketLoadsVariant/BucketLoadsActive/Scale Factor Bucket Empty ==
  note: Dump the bucket load as the bucket angle changes by multiplying the Z force by a factor. This factor gets calculated by the LUT after the bucket angle has dropped below -100 degrees as a way of ensuring the factor is not used prior to the final bucket open move.
  qBucket : Inport
  BucketAngleToBucketLoadPercent : Lookup_n-D  NumberOfTableDimensions=1  BreakpointsForDimension1=[-100 -20]  Table=[1 0]  ExtrapMethod=Clip  UseLastTableValue=on  InternalRulePriority=Speed  RndMeth=Simplest
  Compare To Constant4 : simulink/Logic and Bit Operations/Compare To Constant  relop=<  const=-100  OutDataTypeStr=boolean
  Constant : Constant
  Constant5 : Constant
  Switch6 : Switch  Criteria=u2 > Threshold  SaturateOnIntegerOverflow=off  InputSameDT=off
  Switch7 : Switch  Criteria=u2 > Threshold  SaturateOnIntegerOverflow=off  InputSameDT=off
  Unit Delay3 : UnitDelay  SampleTime=-1
  Scale Load : Outport
  wires:
  Unit Delay3/1 -> Switch6/3
  qBucket/1 -> Compare To Constant4/1, BucketAngleToBucketLoadPercent/1
  BucketAngleToBucketLoadPercent/1 -> Switch7/1
  Constant/1 -> Switch6/1
  Switch6/1 -> Unit Delay3/1, Switch7/2
  Compare To Constant4/1 -> Switch6/2
  Constant5/1 -> Switch7/3
  Switch7/1 -> Scale Load/1

== matlab function Excavator_Complete/Controller/Function Commander/HydraulicCommander ==
  data: swingCmd input; boomCmd input; stickCmd input; bucketCmd input; swingQDmd output; stickHEPr input; stickREPr input; swingSpeed input; boomQDmd output; stickQDmd output; bucketQDmd output; leftPumpDispCmd output; rightPumpDispCmd output; swingMaxQ parameter; boomUpMaxQ parameter; stickOutMaxQ parameter; stickInMaxQ parameter; bucketCloseMaxQ parameter; bucketOpenMaxQ parameter; swingSpoolPos output; boomSpoolPos output; stickSpoolPos output; bucketSpoolPos output; shaftSpeed input; nominalShaftSpeed parameter; minPumpDisp parameter; maxPumpDisp parameter; swingSpeedQGain parameter; swingHighSpeedThreshold parameter
function [swingQDmd, boomQDmd, stickQDmd, bucketQDmd, leftPumpDispCmd, ...
    rightPumpDispCmd, swingSpoolPos, boomSpoolPos, stickSpoolPos, ...
    bucketSpoolPos] = HydraulicCommander( ...
    swingCmd, boomCmd, stickCmd, bucketCmd, stickHEPr, stickREPr, ...
    swingSpeed, swingMaxQ, boomUpMaxQ, stickOutMaxQ, stickInMaxQ, ...
    bucketCloseMaxQ, bucketOpenMaxQ, shaftSpeed, nominalShaftSpeed, ...
    minPumpDisp, maxPumpDisp, swingSpeedQGain, swingHighSpeedThreshold)
%% Initialization
% Flow Rate Demands
swingQDmd = 0; % [lpm]
boomQDmd = 0; % [lpm]
stickQDmd = 0; % [lpm]
bucketQDmd = 0; % [lpm]

% Spool Positions
swingSpoolPos = 0; % [mm]
boomSpoolPos = 0; % [mm]
stickSpoolPos = 0; % [mm]
bucketSpoolPos = 0; % [mm]

% Max Spool Positions
maxPosSpoolPos = 5; % [mm]
maxNegSpoolPos = -5; % [mm]

%% Swing Flow Rate Demand & Spool Position
% Flow Rate
if swingCmd ~= 0
    % Operator command flow rate
    swingOpCmdFlowRate = abs(swingCmd) * swingMaxQ; % [lpm]
  
    % If the swing speed is high or the swing command is opposing the 
    % current speed, use the flow rate directly proportional to the 
    % operator command
    if abs(swingSpeed) > swingHighSpeedThreshold || sign(swingCmd) == sign(swingSpeed)   
        swingQDmd = swingOpCmdFlowRate; % [lpm]
    else
        % Limit the swing flow rate demand based on the current swing speed
        % This limits the flow loss through the swing pressure relief valve
        % during acceleration
        swingSpeedLimitedFlowRate = abs(swingSpeed) * swingSpeedQGain; % [lpm]
        
        % Only use the limited value if it is less than the operator
        % command value
        if swingSpeedLimitedFlowRate < swingOpCmdFlowRate
            swingQDmd = swingSpeedLimitedFlowRate; % [lpm]
        else
            swingQDmd = swingOpCmdFlowRate; % [lpm]
        end
    end 
end

% Spool Position
% Swing Right
if swingCmd > 0
    swingSpoolPos = maxPosSpoolPos; % [mm]
% Swing Left
elseif swingCmd < 0
    swingSpoolPos = maxNegSpoolPos; % [mm]
end

%% Boom Flow Rate Demand & Spool Position
% Boom Up Command Logic - Active Flow
if boomCmd < 0
    boomQDmd = abs(boomCmd) * boomUpMaxQ; % [lpm]
    boomSpoolPos = maxNegSpoolPos; % [mm]
% Boom Down Command Logic - Regenerative Flow
elseif boomCmd > 0
    % For boom down, the valve spool position is varied based on the
    % operator command and there is no pump flow required due to the
    % regenerative flow valve allowing flow from the head end to the rod
    % end during the move. The spool position must be controlled in this 
    % case so that the speed of the boom is proportional to the command. 
    % For boom up, the speed is controlled by limiting the pump flow - but 
    % for boom down, because there is no pump flow, the valve must be used.
    boomSpoolPosFactor = interp1([0 0.10 0.20 0.30 0.40 0.50 0.60 0.70 0.80 0.90 1], ...
                                 [0 0.30 0.45 0.55 0.60 0.70 0.75 0.80 0.85 0.90 1], ...
                                  boomCmd); % [mm]
    boomSpoolPos = maxPosSpoolPos * boomSpoolPosFactor; % [mm]
end

%% Stick Flow Rate Demand & Spool Position
% Stick Out Command Logic - Active Flow
if stickCmd > 0
    stickQDmd = abs(stickCmd) * stickOutMaxQ; % [lpm]
    stickSpoolPos = maxPosSpoolPos; % [mm]
% Stick In Command Logic - Active & Regenerative Flow
elseif stickCmd < 0
    deltaPr = stickREPr - stickHEPr; % [bar]
    if deltaPr > 120
        % When the pressure difference is high, limit the pump flow rate
        % and valve opening to take advantage of the regenerative flow from
        % the rod end. If the valve is opened all the way with a high
        % difference in pressure, the stick velocity will be very high and
        % uncontrolled.  
        stickQDmdFactor = 0.15;
        stickSpoolPosFactor = interp1([0 1], [0 0.55], abs(stickCmd));
    elseif deltaPr > 15
        % When the pressure difference is moderate, start increasing the
        % valve area and pump flow to maintain the velocity.
        stickQDmdFactor = interp1([15 120], [1 0.15], abs(deltaPr));
        stickSpoolPosFactor = interp1([0 1], [0 0.75], abs(stickCmd));
    else
        % When the pressure difference is low, or the head end pressure is
        % higher than the rod end, open the valve completely and allow full
        % pump flow.
        stickQDmdFactor = 1;
        stickSpoolPosFactor = 1;
    end
    % Multiply the maximum flow rate and valve position commands by the
    % factors calculated above to obtain the desired values.
    stickQDmd = abs(stickCmd) * stickInMaxQ * stickQDmdFactor; % [lpm]
    stickSpoolPos = maxNegSpoolPos * stickSpoolPosFactor; % [mm]
end

%% Bucket Flow Rate Demand & Spool Position
% Bucket Open Command Logic - Active Flow
if bucketCmd > 0
    bucketQDmd = abs(bucketCmd) * bucketOpenMaxQ; % [lpm]
    bucketSpoolPos = maxPosSpoolPos; % [mm]
% Bucket Close Command Logic - Active Flow
elseif bucketCmd < 0
    bucketQDmd = abs(bucketCmd) * bucketCloseMaxQ; % [lpm]
    bucketSpoolPos = maxNegSpoolPos; % [mm]
end

%% Pump Distribution
% Max pump flow rate
maxRatedPumpQ = (nominalShaftSpeed * maxPumpDisp)/1000; % [lpm]

% Left Pump: Boom, Stick, Swing
leftPumpQDmd = boomQDmd/2 + stickQDmd/2 + swingQDmd; % [lpm]
% Saturate flow rate demand
if leftPumpQDmd > maxRatedPumpQ
    leftPumpQDmd = maxRatedPumpQ; % [lpm]
end

% Right Pump: Boom, Stick, Bucket
rightPumpQDmd = boomQDmd/2 + stickQDmd/2 + bucketQDmd; % [lpm]
% Saturate flow rate demand
if rightPumpQDmd > maxRatedPumpQ
    rightPumpQDmd = maxRatedPumpQ; % [lpm]
end

%% Left Pump Command
% Convert Flow Rate to Displacement
leftPumpDispCmd = 1000 * (leftPumpQDmd/shaftSpeed); % [cc/rev]
% Saturate displacement command
if leftPumpDispCmd < minPumpDisp
    leftPumpDispCmd = minPumpDisp; % [cc/rev]
elseif leftPumpDispCmd > maxPumpDisp
    leftPumpDispCmd = maxPumpDisp; % [cc/rev]
end

%% Right Pump Command
% Convert Flow Rate to Displacement
rightPumpDispCmd = 1000 * (rightPumpQDmd/shaftSpeed); % [cc/rev]
% Saturate displacement command
if rightPumpDispCmd < minPumpDisp
    rightPumpDispCmd = minPumpDisp; % [cc/rev]
elseif rightPumpDispCmd > maxPumpDisp
    rightPumpDispCmd = maxPumpDisp; % [cc/rev]
end
